simulink model "PMSM_SVPWM_Verify_Discrete"  (R2019a)
settings: Solver=ode3  StartTime=0.0  StopTime=3  FixedStep=1e-6  RelTol=1e-3
InitFcn:
  | %Load Torque
  | Tm = .0;
  | %--- Source
  | Vs = 340; % input voltage
  | 
  | %--- Electric drive
  | P.J = 0.000045; % motor inertia
  | B = 0;
  | %% motor Parameters
  | M.Rs = 11.5;
  | M.Ld = 25e-3;
  | M.Lq = 33.33e-3;
  | M.Lss = (M.Ld + M.Lq)/50;
  | M.AveDiff = (M.Ld+M.Lss+M.Lq+M.Lss)/2;
  | M.HalfDiff = (M.Lq-M.Ld)/2;
  | M.P = 2*8;
  | M.Psir  = 0.119366;
  | M.BaseRpm = 200;
  | M.Id0 = 0;
  | M.Iq0 = 0;
  | M.thm0 = 0;
  | M.is0 = [M.Id0 M.Iq0];
  | 
  | %% current controller
  | D.fpwm = 10000;
  | D.fs = D.fpwm;
  | D.Tpwm = 1/D.fpwm;
  | D.Tdt = 0.00*D.Tpwm; % deadtime
  | D.Ts = 1/D.fs;
  | 
  | D.Tcs = 1/(2*pi*10000); % current sensor bandwidth
  | 
  | %current loop
  | 
  | Ld = M.Ld+M.Lss;
  | R = M.Rs;
  | Lq = M.Lq+M.Lss;
  | Td = Ld/R;
  | Tq = Lq/R;
  | Tres = 4*Tq;
  | alpha = 2.197/Tres;
  | Kpd = alpha*Ld;
  | Kid = alpha*R;
  | Kpq = alpha*Lq;
  | Kiq = alpha*R;
  | 
  | %Kpd = 103.67;
  | %Kid = 348.48;
  | Kpd = 157;
  | Kid = 7.2e4;
  | Kpq = Kpd;
  | Kiq = Kid;
  | 
  | %% speed controller
  | beta = 50;     %30;
  | Kpw = P.J*beta/(1.5*(M.P/2)*M.Psir);
  | Kiw = beta*Kpw;
  | 
  | Kpw = 0.0197;
  | Kiw = 1.24;
undefined symbols (not defined in the file): DiscIntNeverNeededParam
libraries: powerlib x5, cstblocks x3, simulink x2
settings Model: SimulationMode=accelerator  Creator=lovejing  LastModifiedBy=Administrator
settings SolverCC: ZeroCrossAlgorithm=Adaptive
settings DataIOCC: LimitDataPoints=on  SaveFormat=Array  InspectSignalLogs=on  ReturnWorkspaceOutputs=off
settings OptimizationCC: ExpressionDepthLimit=2147483647  EfficientMapNaN2IntZero=off  LifeSpan=inf
settings DebuggingCC: UnderspecifiedInitializationDetection=Classic  MergeDetectMultiDrivingBlocksExec=none  SolverPrmCheckMsg=warning  FcnCallInpInsideContextMsg=warning  StateNameClashWarn=warning  SFUnexpectedBacktrackingDiag=warning  SFNoUnconditionalDefaultTransitionDiag=warning  SFExecutionAtInitializationDiag=none  ArithmeticOperatorsInVariantConditions=warning
settings HardwareCC: ProdBitPerPointer=32  ProdBitPerSizeT=32  ProdBitPerPtrDiffT=32  ProdLargestAtomicFloat=None  ProdIntDivRoundTo=Undefined  ProdEndianess=Unspecified  ProdWordSize=32  ProdHWDeviceType=32-bit Generic  TargetBitPerPointer=64  TargetBitPerSizeT=64  TargetBitPerPtrDiffT=64  TargetLongLongMode=on  TargetIntDivRoundTo=Zero  TargetEndianess=LittleEndian  TargetWordSize=64  TargetHWDeviceType=MATLAB Host  ProdEqTarget=off
settings ModelReferenceCC: PropagateSignalLabelsOutOfModel=off
settings SFSimCC: SimUseLocalCustomCode=off
settings CodeAppCC: MaxIdLength=128
settings GRTTargetCC: TargetLangStandard=C89/C90 (ANSI)  GRTInterface=on
settings ConfigComp: CovMetricSettings=dw  CovHtmlReporting=on  CovSaveCumulativeToWorkspaceVar=on  CovSaveSingleToWorkspaceVar=on  CovExternalEMLEnable=off  CovSFcnEnable=off
settings SimscapeCC: SimscapeNormalizeSystem=off

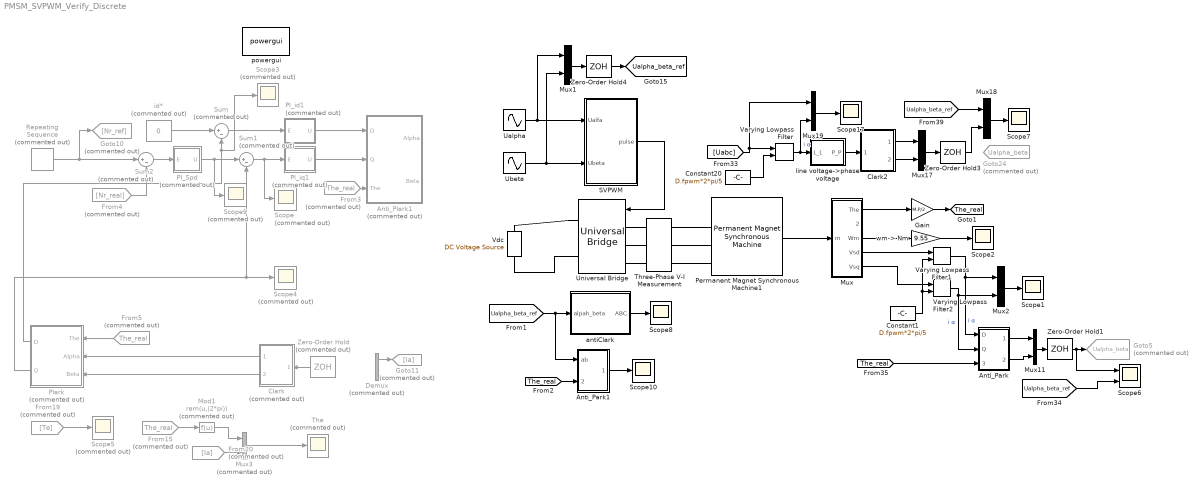
== system PMSM_SVPWM_Verify_Discrete ==
  Anti_Park : Subsystem
  Anti_Park1 : Subsystem
  Anti_Plark1 : Subsystem  Commented=on
  Clark : Subsystem  Commented=on
  Clark2 : Subsystem
  Constant1 : Constant  Value=D.fpwm*2*pi/5
  Constant20 : Constant  Value=D.fpwm*2*pi/5
  Demux : Demux  Commented=on  Outputs=3
  From15 : From  Commented=on  GotoTag=The_real
  From19 : From  Commented=on  GotoTag=Te
  From20 : From  Commented=on  GotoTag=Ia
  From3 : From  Commented=on  GotoTag=The_real
  From4 : From  Commented=on  GotoTag=Nr_real
  From5 : From  Commented=on  GotoTag=The_real
  Gain : Gain  Gain=M.P/2
  Goto10 : Goto  Commented=on  GotoTag=Nr_ref
  Goto11 : Goto  Commented=on  GotoTag=Ia
  Goto24 : Goto  Commented=on  GotoTag=Ualpha_beta  TagVisibility=global
  Goto5 : Goto  Commented=on  GotoTag=Ualpha_beta  TagVisibility=global
  Mod1 : Fcn  Commented=on  Expr=rem(u,(2*pi))
  Mux : Subsystem
  Mux{1..2,11,17..19} (6 alike) : Mux  Inputs=2
  Mux3 : Mux  Commented=on  Inputs=2
  PI_Spd : Subsystem  Commented=on  mask{Kp=Kpw, Ki=Kiw, up_limit=3, low_limit=-3, ts=D.Ts}
      mask prompts: up_limit "upper limit"; low_limit "low limit"; ts "control period"
  PI_id1 : Subsystem  Commented=on  mask{Kp=Kpd, Ki=Kid, up_limit=Vs, low_limit=-Vs, ts=D.Ts}
      mask prompts: up_limit "upper limit"; low_limit "low limit"; ts "control period"
  PI_iq1 : Subsystem  Commented=on  mask{Kp=Kpq, Ki=Kiq, up_limit=Vs, low_limit=-Vs, ts=D.Ts}
      mask prompts: up_limit "upper limit"; low_limit "low limit"; ts "control period"
  Permanent Magnet Synchronous Machine1 : powerlib/Machines/Permanent Magnet Synchronous Machine  NbPhases=3  FluxDistribution=Sinusoidal  RotorType=Salient-pole  MechanicalLoad=Torque Tm  PresetModel=No  ShowDetailedParameters=on  MeasurementBus=off  Resistance=M.Rs  Inductance=8.5e-3  dqInductances=[M.Ld,M.Lq]  La=0.000835  MachineConstant=Flux linkage established by magnets (V.s)  Flux=M.Psir  VoltageCst=64.9518  TorqueCst=0.53715  Flat=120  Mechanical=[0.000045 B M.P/2 Tm]  PolePairs=3  InitialConditions=[0,0, 0,0]  InitialConditions5ph=[0 0 0 0 0 0]  TsPowergui=0  TsBlock=-1  RefAngle=Aligned with phase A axis (original Park)
  Plark : Subsystem  Commented=on
  Repeating Sequence : simulink/Sources/Repeating Sequence  Commented=on  rep_seq_t="[0 1  2 3]"  rep_seq_y="[0  180 180 180]"
  SVPWM : Subsystem  mask{t_pwm=D.Ts, vdc=Vs}
      mask prompts: t_pwm "pwm period"; vdc "bus voltage"
  Scope{,3..5,9} (5 alike) : Scope  Commented=on
  Scope{1..2,7..8,10,17} (6 alike) : Scope
  Scope6 : Scope  NumInputPorts=2
  Sum : Sum  Commented=on  Inputs=|+-
  Sum1 : Sum  Commented=on  Inputs=|+-
  Sum2 : Sum  Commented=on  Inputs=|+-
  The : Scope  Commented=on
  Three-Phase V-I Measurement : powerlib/Measurements/Three-Phase V-I Measurement  VoltageMeasurement=phase-to-phase  SetLabelV=on  LabelV=Uabc  Vpu=off  VpuLL=off  CurrentMeasurement=yes  SetLabelI=on  LabelI=Iabc_m  Ipu=off  Pbase=100e6  Vbase=500e3  OutputType=Complex  PhasorSimulation=off  PSBequivalent=0
      settings: SourceProductName=Simscape Electrical
  Ualpha : Sin  Amplitude=141  Frequency=24*2*pi  SampleTime=0
  Ubeta : Sin  Amplitude=141  Frequency=24*2*pi  Phase=pi/2  SampleTime=0
  Universal Bridge : powerlib/Power Electronics/Universal Bridge  Arms=3  SnubberResistance=1e5  SnubberCapacitance=inf  Device=IGBT / Diodes  Ron=1e-3  Lon=0  ForwardVoltages="[  0  0  ]"  ForwardVoltage=0  GTOparameters=[ 10e-6 , 20e-6 ]  IGBTparameters=[ 1e-6 , 2e-6 ]  Measurements=None  Measurements_2=None  converterType=Rectifier
      settings: SourceProductName=Simscape Electrical
  Varying Lowpass Filter : cstblocks/Linear Parameter Varying/Varying Lowpass Filter  N=1
      settings: SourceProductName=Control System Toolbox
  Varying Lowpass Filter1 : cstblocks/Linear Parameter Varying/Varying Lowpass Filter  N=1
      settings: SourceProductName=Control System Toolbox
  Varying Lowpass Filter2 : cstblocks/Linear Parameter Varying/Varying Lowpass Filter  N=1
      settings: SourceProductName=Control System Toolbox
  "Vdc " : powerlib/Electrical Sources/DC Voltage Source  Amplitude=Vs  Measurements=None
      settings: SourceProductName=Simscape Electrical
  Zero-Order Hold : ZeroOrderHold  Commented=on  SampleTime=D.Ts
  Zero-Order Hold1 : ZeroOrderHold  SampleTime=D.Ts
  Zero-Order Hold3 : ZeroOrderHold  SampleTime=D.Ts
  Zero-Order Hold4 : ZeroOrderHold  SampleTime=D.Ts
  antiClark : Subsystem
  id* : Constant  Commented=on  Value=0
  line voltage->phase voltage : Subsystem
  powergui : powerlib/powergui  Priority=1  SimulationMode=Discrete  SampleTime=1e-6  frequency=60  Iterations=50  frequencyindice=0  Pbase=100e6  ErrMax=1e-4  UnitsV=kV  UnitsW=MW  buscounter=0  FunctionMessages=off  echomessages=off  EnableUseOfTLC=off  CurrentSourceSwitches=on  DisableSnubberDevices=off  DisableRonSwitches=off  DisableVfSwitches=off  DisplayEquations=off  AutomaticDiscreteSolvers=off  SolverType=Tustin/Backward Euler (TBE)  Interpol=off  ExternalGateDelay=off  methode=off  Ts=100  x0status=blocks  SPID=off  SwTol=0  HookPort=off  NonlinearTolerance=0  nMaxIteration=15  ContinueOnMaxIteration=off  RestoreLinks=warning  ResistiveCurrentMeasurement=off  Frange=[0:2:500]  Ylog=off  Xlog=on  ShowGrid=off  save=off  variable=ZData  structure=0  ZoomFFT=off  StartTime=0.0  cycles=1  DisplayStyle=1  fundamental=60  FreqAxis=off  MaxFrequency=1000  frequencyindicesteady=1  RmsSteady=1  display=off
      settings: SourceProductName=Simscape Electrical
  wm-> Nm : Gain  Gain=9.55
  tag scope: The_real=global, Ualpha_beta_ref=global
  wires:
  Clark/1(Alpha) -> Plark/2(Alpha)
  Clark/2(Beta) -> Plark/3(Beta)
  id*/1 -> Sum/1
  Sum/1 -> PI_id1/1(E)
  Sum1/1 -> PI_iq1/1(E), Scope/1
  PI_iq1/1(U) -> Anti_Plark1/2(Q)
  Mux/3(Wm) -> wm-> Nm/1
  wm-> Nm/1 -> Scope2/1
  Mux/1(The) -> Gain/1
  SVPWM/1(pulse) -> Universal Bridge/1
  Plark/2(Q) -> Sum1/2, Scope4/1
  PI_Spd/1(U) -> Scope9/1, Sum1/1
  PI_id1/1(U) -> Anti_Plark1/1(D)
  From15/1 -> Mod1/1
  Mod1/1 -> Mux3/1
  Mux3/1 -> The/1
  Plark/1(D) -> Scope3/1, Sum/2
  Repeating Sequence/1 -> Sum2/1, Goto10/1
  From19/1 -> Scope5/1
  Demux/1 -> Goto11/1
  From5/1 -> Plark/1(The)
  From20/1 -> Mux3/2
  From3/1 -> Anti_Plark1/3(The)
  Sum2/1 -> PI_Spd/1(E)
  From4/1 -> Sum2/2
  Zero-Order Hold/1 -> Clark/1(ABC)
  Mux17/1 -> Zero-Order Hold3/1
  Zero-Order Hold3/1 -> Mux18/2
  Clark2/2(Beta) -> Mux17/2
  Clark2/1(Alpha) -> Mux17/1
  Constant20/1 -> Varying Lowpass Filter/2
  Varying Lowpass Filter/1 -> Mux19/2, line voltage->phase voltage/1(L_L)  "i α"
  Mux19/1 -> Scope17/1
  [Ualpha_beta_ref] -> Mux18/1
  [Uabc] -> Varying Lowpass Filter/1, Mux19/1
  line voltage->phase voltage/1(P_P) -> Clark2/1(ABC)
  Mux18/1 -> Scope7/1
  Permanent Magnet Synchronous Machine1/1 -> Mux/1(m)
  Gain/1 -> [The_real]
  Anti_Park/1(Alpha) -> Mux11/1
  [The_real] -> Anti_Park/3(The)
  Mux11/1 -> Zero-Order Hold1/1
  Zero-Order Hold1/1 -> Scope6/1, Goto5/1
  Anti_Park/2(Beta) -> Mux11/2
  [Ualpha_beta_ref] -> Scope6/2
  Ubeta/1 -> Mux1/2, SVPWM/2(Ubeta)
  Zero-Order Hold4/1 -> [Ualpha_beta_ref]
  Ualpha/1 -> Mux1/1, SVPWM/1(Ualfa)
  Mux1/1 -> Zero-Order Hold4/1
  Mux/4(Vsd) -> Varying Lowpass Filter1/1
  Mux/5(Vsq) -> Varying Lowpass Filter2/1
  Varying Lowpass Filter1/1 -> Mux2/1, Anti_Park/1(D)  "i α"
  Varying Lowpass Filter2/1 -> Anti_Park/2(Q), Mux2/2  "i α"
  Constant1/1 -> Varying Lowpass Filter1/2, Varying Lowpass Filter2/2
  Mux2/1 -> Scope1/1
  [Ualpha_beta_ref] -> Anti_Park1/1(ab), antiClark/1(alpah_beta)
  antiClark/1(ABC) -> Scope8/1
  Anti_Park1/1(DQ) -> Scope10/1
  [The_real] -> Anti_Park1/2(The)
  connections:
  "Vdc "/LConn1 -- Universal Bridge/RConn2
  Universal Bridge/RConn1 -- "Vdc "/RConn1
  Universal Bridge/LConn1 -- Three-Phase V-I Measurement/LConn1
  Three-Phase V-I Measurement/RConn1 -- Permanent Magnet Synchronous Machine1/LConn1
  Universal Bridge/LConn2 -- Three-Phase V-I Measurement/LConn2
  Three-Phase V-I Measurement/RConn2 -- Permanent Magnet Synchronous Machine1/LConn2
  Universal Bridge/LConn3 -- Three-Phase V-I Measurement/LConn3
  Three-Phase V-I Measurement/RConn3 -- Permanent Magnet Synchronous Machine1/LConn3

== system PMSM_SVPWM_Verify_Discrete/Anti_Park ==
  D : Inport
  Q : Inport  Port=2
  The : Inport  Port=3
  Mux : Mux  Inputs=3
  alpha : Fcn  Expr=u(1)*cos(u(3))-u(2)*sin(u(3))
  beta : Fcn  Expr=u(1)*sin(u(3))+u(2)*cos(u(3))
  Alpha : Outport
  Beta : Outport  Port=2
  wires:
  beta/1 -> Beta/1
  Mux/1 -> alpha/1, beta/1
  D/1 -> Mux/1
  The/1 -> Mux/3
  Q/1 -> Mux/2
  alpha/1 -> Alpha/1

== system PMSM_SVPWM_Verify_Discrete/Anti_Park1 ==
  ab : Inport
  The : Inport  Port=2
  D : Fcn  Expr=u(1)*cos(u(3))+u(2)*sin(u(3))
  Mux : Mux  Inputs=2
  Mux1 : Mux  Inputs=2
  Q : Fcn  Expr=-u(1)*sin(u(3))+u(2)*cos(u(3))
  DQ : Outport
  wires:
  ab/1 -> Mux/1
  Mux/1 -> Q/1, D/1
  The/1 -> Mux/2
  Mux1/1 -> DQ/1
  D/1 -> Mux1/1
  Q/1 -> Mux1/2

== system PMSM_SVPWM_Verify_Discrete/Anti_Plark1 ==
  D : Inport
  Q : Inport  Port=2
  The : Inport  Port=3
  Mux : Mux  Inputs=3
  alpha : Fcn  Expr=u(1)*cos(u(3))-u(2)*sin(u(3))
  beta : Fcn  Expr=u(1)*sin(u(3))+u(2)*cos(u(3))
  Alpha : Outport
  Beta : Outport  Port=2
  wires:
  alpha/1 -> Alpha/1
  Q/1 -> Mux/2
  The/1 -> Mux/3
  D/1 -> Mux/1
  Mux/1 -> beta/1, alpha/1
  beta/1 -> Beta/1

== system PMSM_SVPWM_Verify_Discrete/Clark ==
  ABC : Inport
  alpha : Fcn  Expr=(u(1)-0.5*(u(2)+u(3)))*2/3
  beta : Fcn  Expr=sqrt(3)/2*(u(2)-u(3))*2/3
  Alpha : Outport
  Beta : Outport  Port=2
  wires:
  alpha/1 -> Alpha/1
  ABC/1 -> beta/1, alpha/1
  beta/1 -> Beta/1

== system PMSM_SVPWM_Verify_Discrete/Clark2 ==
  ABC : Inport
  alpha : Fcn  Expr=(u(1)-0.5*(u(2)+u(3)))*2/3
  beta : Fcn  Expr=sqrt(3)/2*(u(2)-u(3))*2/3
  Alpha : Outport
  Beta : Outport  Port=2
  wires:
  alpha/1 -> Alpha/1
  ABC/1 -> beta/1, alpha/1
  beta/1 -> Beta/1

== system PMSM_SVPWM_Verify_Discrete/Mux ==
  m : Inport
  Bus Selector : BusSelector  OutputSignals=Stator current is_a (A),Stator current is_b (A),Stator current is_c (A)
  Bus Selector1 : BusSelector  OutputSignals=Rotor speed wm (rad/s),Rotor angle thetam (rad),Stator voltage Vs_d (V),Stator voltage Vs_q (V)
  Mux : Mux  Inputs=3
  The : Outport
  Iabc : Outport  Port=2
  Wm : Outport  Port=3
  Vsd : Outport  Port=4
  Vsq : Outport  Port=5
  wires:
  Bus Selector1/1 -> Wm/1  "<Rotor speed wm (rad/s)>"
  Bus Selector1/2 -> The/1  "<Rotor angle thetam (rad)>"
  m/1 -> Bus Selector/1, Bus Selector1/1
  Bus Selector/2 -> Mux/2  "<Stator current is_b (A)>"
  Bus Selector/3 -> Mux/3  "<Stator current is_c (A)>"
  Bus Selector/1 -> Mux/1  "<Stator current is_a (A)>"
  Mux/1 -> Iabc/1
  Bus Selector1/3 -> Vsd/1  "<Stator voltage Vs_d (V)>"
  Bus Selector1/4 -> Vsq/1  "<Stator voltage Vs_q (V)>"

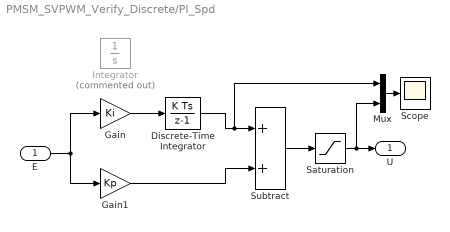
== system PMSM_SVPWM_Verify_Discrete/PI_Spd ==
  E : Inport  SampleTime=ts
  Discrete-Time Integrator : DiscreteIntegrator  SampleTime=ts  LimitOutput=on  UpperSaturationLimit=up_limit  LowerSaturationLimit=low_limit  ICPrevOutput=DiscIntNeverNeededParam  ICPrevScaledInput=DiscIntNeverNeededParam
  Gain : Gain  Gain=Ki
  Gain1 : Gain  Gain=Kp
  Integrator : Integrator  Commented=on
  Mux : Mux  Inputs=2
  Saturation : Saturate  UpperLimit=up_limit  LowerLimit=low_limit
  Scope : Scope
  Subtract : Sum  OutDataTypeStr=Inherit: Same as accumulator
  U : Outport  SampleTime=ts
  wires:
  E/1 -> Gain/1, Gain1/1
  Discrete-Time Integrator/1 -> Mux/1, Subtract/1
  Gain1/1 -> Subtract/2
  Subtract/1 -> Saturation/1
  Saturation/1 -> Mux/2, U/1
  Gain/1 -> Discrete-Time Integrator/1
  Mux/1 -> Scope/1

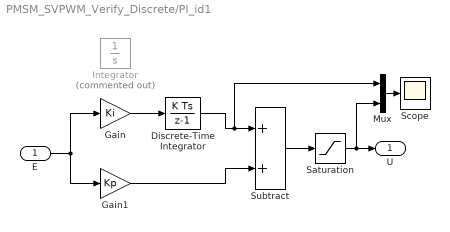
== system PMSM_SVPWM_Verify_Discrete/PI_id1 ==
  E : Inport  SampleTime=ts
  Discrete-Time Integrator : DiscreteIntegrator  SampleTime=ts  LimitOutput=on  UpperSaturationLimit=up_limit  LowerSaturationLimit=low_limit  ICPrevOutput=DiscIntNeverNeededParam  ICPrevScaledInput=DiscIntNeverNeededParam
  Gain : Gain  Gain=Ki
  Gain1 : Gain  Gain=Kp
  Integrator : Integrator  Commented=on
  Mux : Mux  Inputs=2
  Saturation : Saturate  UpperLimit=up_limit  LowerLimit=low_limit
  Scope : Scope
  Subtract : Sum
  U : Outport  SampleTime=ts
  wires:
  Mux/1 -> Scope/1
  Gain/1 -> Discrete-Time Integrator/1
  Saturation/1 -> U/1, Mux/2
  Subtract/1 -> Saturation/1
  Gain1/1 -> Subtract/2
  Discrete-Time Integrator/1 -> Subtract/1, Mux/1
  E/1 -> Gain1/1, Gain/1

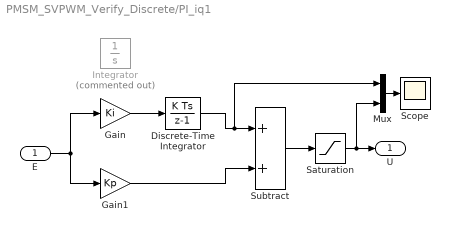
== system PMSM_SVPWM_Verify_Discrete/PI_iq1 ==
  E : Inport  SampleTime=ts
  Discrete-Time Integrator : DiscreteIntegrator  SampleTime=ts  LimitOutput=on  UpperSaturationLimit=up_limit  LowerSaturationLimit=low_limit  ICPrevOutput=DiscIntNeverNeededParam  ICPrevScaledInput=DiscIntNeverNeededParam
  Gain : Gain  Gain=Ki
  Gain1 : Gain  Gain=Kp
  Integrator : Integrator  Commented=on
  Mux : Mux  Inputs=2
  Saturation : Saturate  UpperLimit=up_limit  LowerLimit=low_limit
  Scope : Scope
  Subtract : Sum
  U : Outport  SampleTime=ts
  wires:
  E/1 -> Gain/1, Gain1/1
  Discrete-Time Integrator/1 -> Mux/1, Subtract/1
  Gain1/1 -> Subtract/2
  Subtract/1 -> Saturation/1
  Saturation/1 -> Mux/2, U/1
  Gain/1 -> Discrete-Time Integrator/1
  Mux/1 -> Scope/1

== system PMSM_SVPWM_Verify_Discrete/Plark ==
  The : Inport
  Alpha : Inport  Port=2
  Beta : Inport  Port=3
  DQ_AB : Scope
  Mux : Mux  Inputs=3
  Mux2 : Mux
  d : Fcn  Expr=u(1)*cos(u(3))+u(2)*sin(u(3))
  q : Fcn  Expr=-u(1)*sin(u(3))+u(2)*cos(u(3))
  D : Outport
  Q : Outport  Port=2
  wires:
  d/1 -> Mux2/3, D/1
  Beta/1 -> Mux/2
  The/1 -> Mux2/2, Mux/3
  Alpha/1 -> Mux2/1, Mux/1
  Mux/1 -> q/1, d/1
  q/1 -> Mux2/4, Q/1
  Mux2/1 -> DQ_AB/1

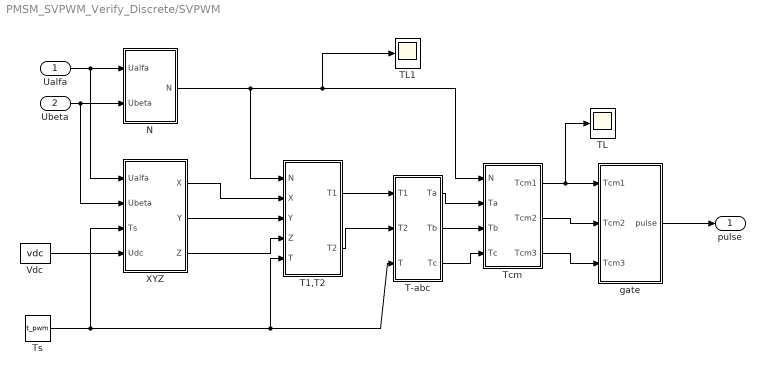
== system PMSM_SVPWM_Verify_Discrete/SVPWM ==
  Ualfa : Inport
  Ubeta : Inport  Port=2
  N : Subsystem
  T-abc : Subsystem
  T1,T2 : Subsystem
  TL : Scope
  TL1 : Scope
  Tcm : Subsystem
  Ts : Constant  Value=t_pwm  SampleTime=-1
  Vdc : Constant  Value=vdc
  XYZ : Subsystem
  gate : Subsystem
  pulse : Outport
  wires:
  Tcm/1(Tcm1) -> gate/1(Tcm1), TL/1
  T-abc/2(Tb) -> Tcm/3(Tb)
  T-abc/1(Ta) -> Tcm/2(Ta)
  T-abc/3(Tc) -> Tcm/4(Tc)
  T1,T2/1(T1) -> T-abc/1(T1)
  T1,T2/2(T2) -> T-abc/2(T2)
  XYZ/2(Y) -> T1,T2/3(Y)
  XYZ/1(X) -> T1,T2/2(X)
  XYZ/3(Z) -> T1,T2/4(Z)
  N/1(N) -> T1,T2/1(N), TL1/1, Tcm/1(N)
  Ts/1 -> T1,T2/5(T), T-abc/3(T), XYZ/3(Ts)
  gate/1(pulse) -> pulse/1
  Ualfa/1 -> N/1(Ualfa), XYZ/1(Ualfa)
  Ubeta/1 -> N/2(Ubeta), XYZ/2(Ubeta)
  Vdc/1 -> XYZ/4(Udc)
  Tcm/2(Tcm2) -> gate/2(Tcm2)
  Tcm/3(Tcm3) -> gate/3(Tcm3)

== system PMSM_SVPWM_Verify_Discrete/antiClark ==
  alpah_beta : Inport
  Mux : Mux  Inputs=3
  alpha : Fcn  Expr=(u(1))
  beta : Fcn  Expr=sqrt(3)/2*u(2)-u(1)/2
  beta1 : Fcn  Expr=-sqrt(3)/2*u(2)-u(1)/2
  ABC : Outport
  wires:
  alpah_beta/1 -> alpha/1, beta1/1, beta/1
  Mux/1 -> ABC/1
  beta/1 -> Mux/2
  alpha/1 -> Mux/1
  beta1/1 -> Mux/3

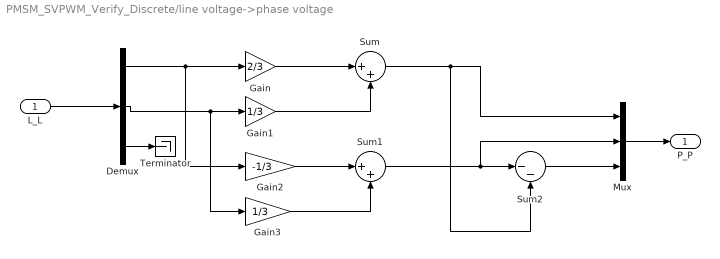
== system PMSM_SVPWM_Verify_Discrete/line voltage->phase voltage ==
  L_L : Inport
  Demux : Demux  Outputs=3
  Gain : Gain  Gain=2/3
  Gain1 : Gain  Gain=1/3
  Gain2 : Gain  Gain=-1/3
  Gain3 : Gain  Gain=1/3
  Mux : Mux  Inputs=3
  Sum : Sum  Inputs=|++
  Sum1 : Sum  Inputs=|++
  Sum2 : Sum  Inputs=|--
  Terminator : Terminator
  P_P : Outport
  wires:
  Demux/2 -> Gain3/1, Gain1/1
  Demux/1 -> Gain2/1, Gain/1
  Gain/1 -> Sum/1
  Gain1/1 -> Sum/2
  Gain2/1 -> Sum1/1
  Gain3/1 -> Sum1/2
  Sum/1 -> Sum2/2, Mux/1
  Sum2/1 -> Mux/3
  Sum1/1 -> Mux/2, Sum2/1
  Mux/1 -> P_P/1
  L_L/1 -> Demux/1
  Demux/3 -> Terminator/1

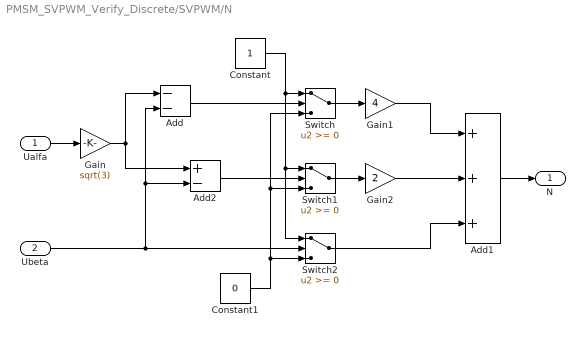
== system PMSM_SVPWM_Verify_Discrete/SVPWM/N ==
  Ualfa : Inport
  Ubeta : Inport  Port=2
  Add : Sum  Inputs=--
  Add1 : Sum  Inputs=+++
  Add2 : Sum  Inputs=+-
  Constant : Constant
  Constant1 : Constant  Value=0
  Gain : Gain  Gain=sqrt(3)
  Gain1 : Gain  Gain=4
  Gain2 : Gain  Gain=2
  Switch : Switch
  Switch1 : Switch
  Switch2 : Switch
  N : Outport
  wires:
  Ualfa/1 -> Gain/1
  Add1/1 -> N/1
  Switch/1 -> Gain1/1
  Add/1 -> Switch/2
  Gain/1 -> Add/1, Add2/1
  Ubeta/1 -> Switch2/2, Add/2, Add2/2
  Gain1/1 -> Add1/1
  Switch2/1 -> Add1/3
  Add2/1 -> Switch1/2
  Switch1/1 -> Gain2/1
  Gain2/1 -> Add1/2
  Constant/1 -> Switch2/1, Switch1/1, Switch/1
  Constant1/1 -> Switch/3, Switch1/3, Switch2/3

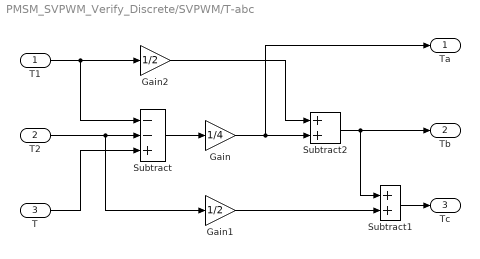
== system PMSM_SVPWM_Verify_Discrete/SVPWM/T-abc ==
  T1 : Inport
  T2 : Inport  Port=2
  T : Inport  Port=3
  Gain : Gain  Gain=1/4
  Gain1 : Gain  Gain=1/2
  Gain2 : Gain  Gain=1/2
  Subtract : Sum  Inputs=--+
  Subtract1 : Sum
  Subtract2 : Sum
  Ta : Outport
  Tb : Outport  Port=2
  Tc : Outport  Port=3
  wires:
  T2/1 -> Subtract/2, Gain1/1
  T1/1 -> Subtract/1, Gain2/1
  T/1 -> Subtract/3
  Subtract/1 -> Gain/1
  Gain/1 -> Ta/1, Subtract2/2
  Gain2/1 -> Subtract2/1
  Subtract2/1 -> Tb/1, Subtract1/1
  Subtract1/1 -> Tc/1
  Gain1/1 -> Subtract1/2

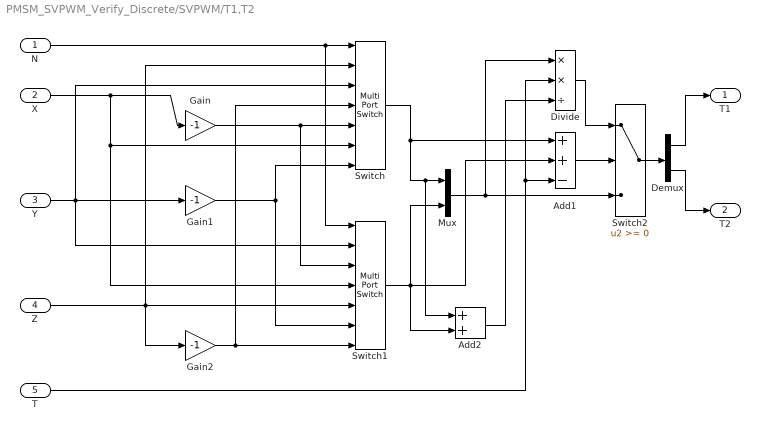
== system PMSM_SVPWM_Verify_Discrete/SVPWM/T1,T2 ==
  N : Inport
  X : Inport  Port=2
  Y : Inport  Port=3
  Z : Inport  Port=4
  T : Inport  Port=5
  Add1 : Sum  Inputs=++-
  Add2 : Sum
  Demux : Demux  Outputs=2
  Divide : Product  Inputs=**/
  Gain : Gain  Gain=-1
  Gain1 : Gain  Gain=-1
  Gain2 : Gain  Gain=-1
  Mux : Mux  Inputs=2
  Switch : MultiPortSwitch  Inputs=6  DiagnosticForDefault=None
  Switch1 : MultiPortSwitch  Inputs=6  DiagnosticForDefault=None
  Switch2 : Switch
  T1 : Outport
  T2 : Outport  Port=2
  wires:
  Y/1 -> Switch/3, Gain1/1, Switch1/2
  Z/1 -> Switch/2, Switch1/5, Gain2/1
  X/1 -> Gain/1, Switch1/4, Switch/6
  Gain/1 -> Switch/5, Switch1/3
  Gain2/1 -> Switch/4, Switch1/7
  Gain1/1 -> Switch1/6, Switch/7
  Switch/1 -> Add1/1, Mux/1, Add2/1
  Switch1/1 -> Mux/2, Add1/2, Add2/2
  Mux/1 -> Divide/1, Switch2/3
  Switch2/1 -> Demux/1
  Demux/1 -> T1/1
  Demux/2 -> T2/1
  Add1/1 -> Switch2/2
  T/1 -> Add1/3, Divide/2
  Divide/1 -> Switch2/1
  Add2/1 -> Divide/3
  N/1 -> Switch/1, Switch1/1

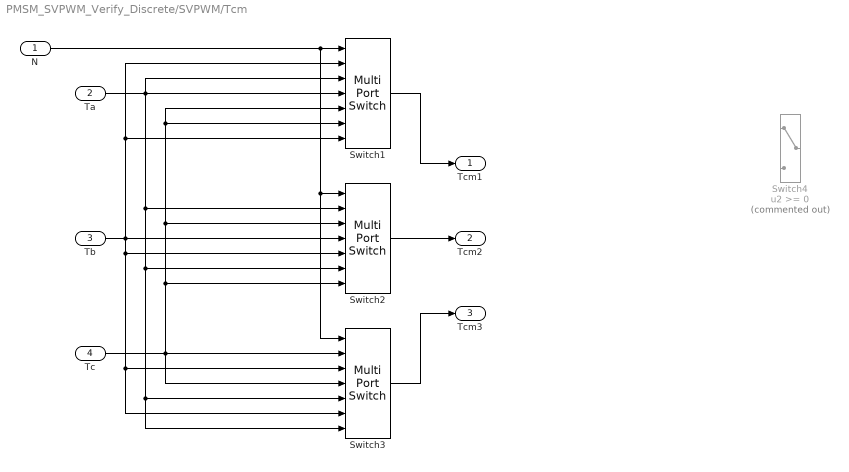
== system PMSM_SVPWM_Verify_Discrete/SVPWM/Tcm ==
  N : Inport
  Ta : Inport  Port=2
  Tb : Inport  Port=3
  Tc : Inport  Port=4
  Switch1 : MultiPortSwitch  Inputs=6  DiagnosticForDefault=None
  Switch2 : MultiPortSwitch  Inputs=6  DiagnosticForDefault=None
  Switch3 : MultiPortSwitch  Inputs=6  DiagnosticForDefault=None
  Switch4 : Switch  Commented=on
  Tcm1 : Outport
  Tcm2 : Outport  Port=2
  Tcm3 : Outport  Port=3
  wires:
  Switch2/1 -> Tcm2/1
  Switch3/1 -> Tcm3/1
  Switch1/1 -> Tcm1/1
  Tb/1 -> Switch2/4, Switch2/5, Switch3/3, Switch3/6, Switch1/2, Switch1/7
  Tc/1 -> Switch3/2, Switch3/4, Switch2/3, Switch1/5, Switch1/6, Switch2/7
  Ta/1 -> Switch1/4, Switch1/3, Switch2/2, Switch2/6, Switch3/5, Switch3/7
  N/1 -> Switch1/1, Switch2/1, Switch3/1

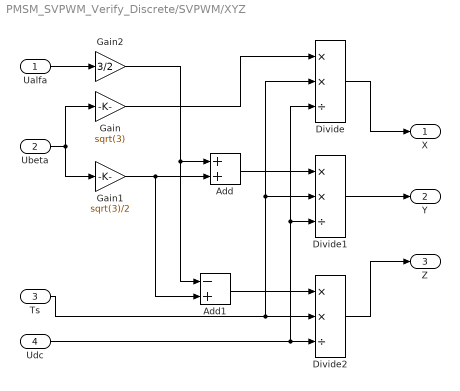
== system PMSM_SVPWM_Verify_Discrete/SVPWM/XYZ ==
  Ualfa : Inport
  Ubeta : Inport  Port=2
  Ts : Inport  Port=3
  Udc : Inport  Port=4
  Add : Sum
  Add1 : Sum  Inputs=-+
  Divide : Product  Inputs=**/
  Divide1 : Product  Inputs=**/
  Divide2 : Product  Inputs=**/
  Gain : Gain  Gain=sqrt(3)
  Gain1 : Gain  Gain=sqrt(3)/2
  Gain2 : Gain  Gain=3/2
  X : Outport
  Y : Outport  Port=2
  Z : Outport  Port=3
  wires:
  Divide1/1 -> Y/1
  Divide/1 -> X/1
  Divide2/1 -> Z/1
  Ts/1 -> Divide2/2, Divide1/2, Divide/2
  Udc/1 -> Divide2/3, Divide1/3, Divide/3
  Ubeta/1 -> Gain/1, Gain1/1
  Ualfa/1 -> Gain2/1
  Gain/1 -> Divide/1
  Add/1 -> Divide1/1
  Gain1/1 -> Add/2, Add1/2
  Gain2/1 -> Add1/1, Add/1
  Add1/1 -> Divide2/1

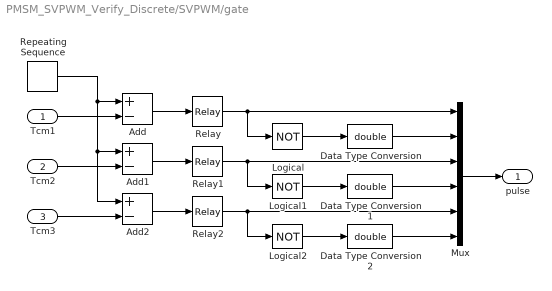
== system PMSM_SVPWM_Verify_Discrete/SVPWM/gate ==
  Tcm1 : Inport
  Tcm2 : Inport  Port=2
  Tcm3 : Inport  Port=3
  Add : Sum  Inputs=+-
  Add1 : Sum  Inputs=+-
  Add2 : Sum  Inputs=+-
  Data Type Conversion : DataTypeConversion  OutDataTypeStr=double
  Data Type Conversion1 : DataTypeConversion  OutDataTypeStr=double
  Data Type Conversion2 : DataTypeConversion  OutDataTypeStr=double
  Logical : Logic  Operator=NOT  AllPortsSameDT=off  OutDataTypeStr=boolean
  Logical1 : Logic  Operator=NOT  AllPortsSameDT=off  OutDataTypeStr=boolean
  Logical2 : Logic  Operator=NOT  AllPortsSameDT=off  OutDataTypeStr=boolean
  Mux : Mux  Inputs=6
  Relay : Relay
  Relay1 : Relay
  Relay2 : Relay
  Repeating Sequence : simulink/Sources/Repeating Sequence  rep_seq_t=[0 t_pwm/2 t_pwm]  rep_seq_y=[0 t_pwm/2 0]
  pulse : Outport
  wires:
  Tcm1/1 -> Add/2
  Tcm2/1 -> Add1/2
  Tcm3/1 -> Add2/2
  Repeating Sequence/1 -> Add2/1, Add1/1, Add/1
  Add2/1 -> Relay2/1
  Add1/1 -> Relay1/1
  Add/1 -> Relay/1
  Relay/1 -> Mux/1, Logical/1
  Relay1/1 -> Mux/3, Logical1/1
  Relay2/1 -> Mux/5, Logical2/1
  Data Type Conversion/1 -> Mux/2
  Logical/1 -> Data Type Conversion/1
  Data Type Conversion1/1 -> Mux/4
  Logical1/1 -> Data Type Conversion1/1
  Data Type Conversion2/1 -> Mux/6
  Logical2/1 -> Data Type Conversion2/1
  Mux/1 -> pulse/1
